simulink model "first1"  (R2023b)
settings: Solver=FixedStepAuto  StartTime=0.0  StopTime=10  FixedStep=0.0001  RelTol=1e-3
values from neighbouring files (symbols this model uses):
  A = [-1 0 0 0 ... (first row only)    [untitled.m]    (also in untitled2.m)
  B = [0;1;0;1]    [untitled.m]    (also in untitled2.m)
  K = -Y*pinv(P)    [untitled.m]    (also in untitled2.m)
undefined symbols (not defined in the file or in its folder): C, K1, K2, x0
settings Model: Creator=evdokiiagalkina  LastModifiedBy=evdokiiagalkina

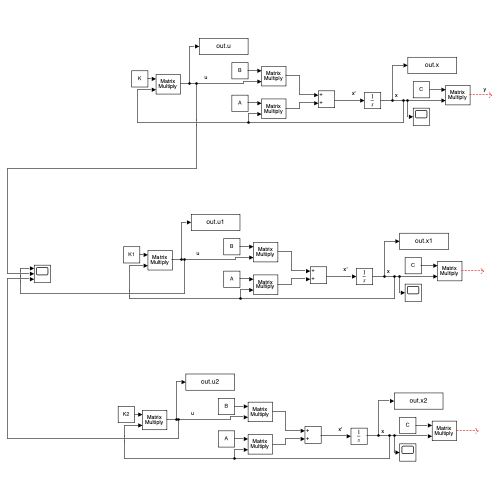
[thumbnail: Simulink's stored preview of the top-level diagram]
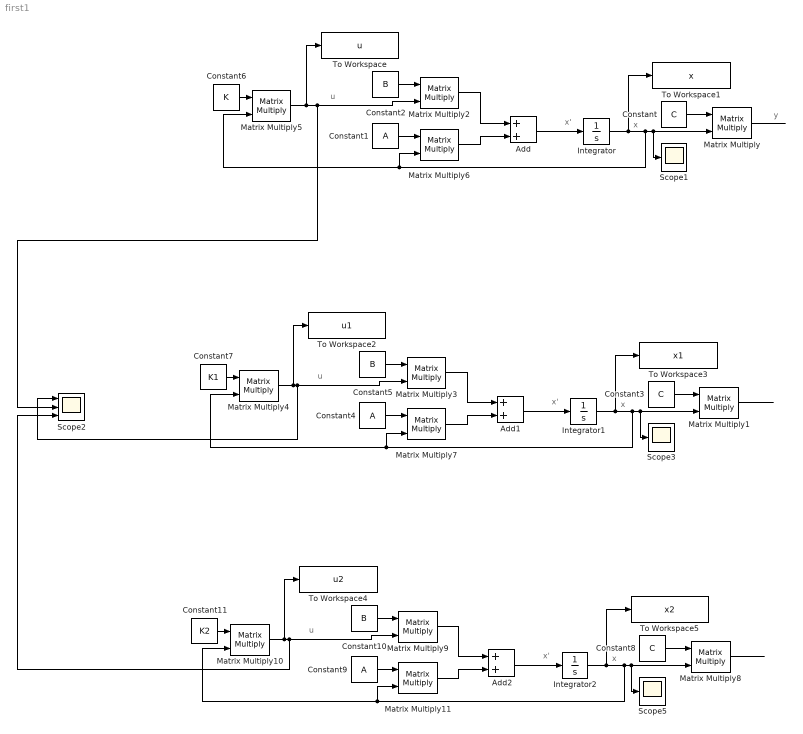
== system first1 ==
  note: u
  note: y
  note: x'
  note: x
  note: x'
  note: u
  note: x
  note: x'
  note: u
  note: x
  Add : Sum
  Add1 : Sum
  Add2 : Sum
  Constant : Constant  Value=C
  Constant1 : Constant  Value=A
  Constant10 : Constant  Value=B
  Constant11 : Constant  Value=K2  VectorParams1D=off
  Constant2 : Constant  Value=B
  Constant3 : Constant  Value=C
  Constant4 : Constant  Value=A
  Constant5 : Constant  Value=B
  Constant6 : Constant  Value=K  VectorParams1D=off
  Constant7 : Constant  Value=K1  VectorParams1D=off
  Constant8 : Constant  Value=C
  Constant9 : Constant  Value=A
  Integrator : Integrator  InitialCondition=x0  IgnoreLimit=on
  Integrator1 : Integrator  InitialCondition=x0  IgnoreLimit=on
  Integrator2 : Integrator  InitialCondition=x0  IgnoreLimit=on
  Matrix Multiply{,1..11} (12 alike) : Product  Multiplication=Matrix(*)
  Scope1 : Scope
  Scope2 : Scope  NumInputPorts=3
  Scope3 : Scope
  Scope5 : Scope
  To Workspace : ToWorkspace  VariableName=u  SaveFormat=Timeseries  SampleTime=-1
  To Workspace1 : ToWorkspace  VariableName=x  SaveFormat=Timeseries  SampleTime=-1
  To Workspace2 : ToWorkspace  VariableName=u1  SaveFormat=Timeseries  SampleTime=-1
  To Workspace3 : ToWorkspace  VariableName=x1  SaveFormat=Timeseries  SampleTime=-1
  To Workspace4 : ToWorkspace  VariableName=u2  SaveFormat=Timeseries  SampleTime=-1
  To Workspace5 : ToWorkspace  VariableName=x2  SaveFormat=Timeseries  SampleTime=-1
  wires:
  Integrator/1 -> To Workspace1/1, Matrix Multiply6/2, Matrix Multiply5/2, Scope1/1, Matrix Multiply/2
  Matrix Multiply/1 -> ?
  Matrix Multiply6/1 -> Add/2
  Matrix Multiply2/1 -> Add/1
  Constant/1 -> Matrix Multiply/1
  Constant6/1 -> Matrix Multiply5/1
  Constant2/1 -> Matrix Multiply2/1
  Matrix Multiply5/1 -> Scope2/2, Matrix Multiply2/2, To Workspace/1
  Constant1/1 -> Matrix Multiply6/1
  Add/1 -> Integrator/1
  Constant5/1 -> Matrix Multiply3/1
  Matrix Multiply3/1 -> Add1/1
  Integrator1/1 -> To Workspace3/1, Matrix Multiply7/2, Matrix Multiply4/2, Scope3/1, Matrix Multiply1/2
  Constant7/1 -> Matrix Multiply4/1
  Matrix Multiply7/1 -> Add1/2
  Constant3/1 -> Matrix Multiply1/1
  Matrix Multiply1/1 -> ?
  Add1/1 -> Integrator1/1
  Matrix Multiply4/1 -> Matrix Multiply3/2, Scope2/1, To Workspace2/1
  Constant4/1 -> Matrix Multiply7/1
  Constant10/1 -> Matrix Multiply9/1
  Matrix Multiply9/1 -> Add2/1
  Integrator2/1 -> To Workspace5/1, Matrix Multiply11/2, Matrix Multiply10/2, Scope5/1, Matrix Multiply8/2
  Constant11/1 -> Matrix Multiply10/1
  Matrix Multiply11/1 -> Add2/2
  Constant8/1 -> Matrix Multiply8/1
  Matrix Multiply8/1 -> ?
  Add2/1 -> Integrator2/1
  Matrix Multiply10/1 -> Scope2/3, Matrix Multiply9/2, To Workspace4/1
  Constant9/1 -> Matrix Multiply11/1
